simulink model "sfcndemo_dsfunc"  (Simulink 7.6)
settings: Solver=FixedStepDiscrete  StartTime=0.0  StopTime=10.0  RelTol=1e-3
Description:
  | Discrete-Time State-Space C-MEX S-function
settings Model: Creator=The MathWorks Inc.  ExtModeTrigMode=oneshot  ExtModeArmWhenConnect=off  ExtModeAutoUpdateStatusClock=off
settings DataIOCC: LimitDataPoints=off
settings OptimizationCC: BlockReduction=off  BooleanDataType=off  InlineInvariantSignals=on  InitFltsAndDblsToZero=on
settings DebuggingCC: SaveWithParameterizedLinksMsg=none  SignalResolutionControl=TryResolveAllWithWarning  SolverPrmCheckMsg=none  MultiTaskDSMMsg=warning  MultiTaskCondExecSysMsg=none
settings HardwareCC: TargetUnknown=on
settings RTWCC: IncludeERTFirstTime=on
settings CodeAppCC: CustomSymbolStrFcn=$F$N$M
settings GRTTargetCC: TargetFcnLib=ansi_tfl_tmw.mat

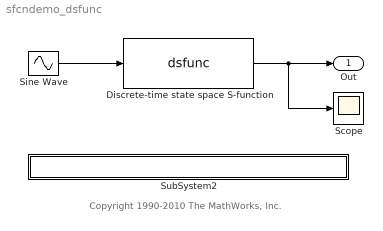
== system sfcndemo_dsfunc ==
  note: Copyright 1990-2010 The MathWorks, Inc.
  "Discrete-time state space S-function " : S-Function  FunctionName=dsfunc  EnableBusSupport=off
      mask Type: S-function: dsfunc
      mask Description: This is a S-function which does the discrete state space system.
      mask Display: disp('x(n+1) = Ax(n) + Bu(n)\n y(n)     = Cx(n) + Du(n) ');
  Scope : Scope
      settings: TimeRange=10  YMin=-70  YMax=65
  Sine Wave : Sin  Amplitude=[1 2]  SampleTime=0
  SubSystem2 : Subsystem  mask{filename=dsfunc.c}
      mask init:
      | x=sfundemo_maskdisp;
      settings: AttributesFormatString=\n  OpenFcn=sfundemo_openfcn
      mask Display: disp(x);
  Out : Outport  InitialOutput=0
  wires:
  Sine Wave/1 -> "Discrete-time state space S-function "/1
  "Discrete-time state space S-function "/1 -> Out/1, Scope/1

== system sfcndemo_dsfunc/SubSystem2 ==
